simulink model "controladorNovo2015"  (R2015b)
settings: Solver=FixedStepDiscrete  SolverMode=SingleTasking  StartTime=0.0  StopTime=tmax  FixedStep=h  RelTol=1e-3
values from neighbouring files (symbols this model uses):
  G = [1; 1]    [init.m]    (also in initTemp.m = tf(N, D))
  h = 0.01    [init.m]    (also in initTemp.m)
  Qn = 0.01    [init.m]
  R = 0.01    [init.m]
  x0 = [1;1]    [init.m]
undefined symbols (not defined in the file or in its folder): C, Cd, gama, H, phi
libraries: simulink x1, dspsrcs4 x1
settings Model: Creator=Raposo  LastModifiedBy=lucasperovani
settings DataIOCC: LimitDataPoints=off
settings DebuggingCC: SFUnexpectedBacktrackingDiag=error  SFNoUnconditionalDefaultTransitionDiag=error
settings HardwareCC: ProdWordSize=32  ProdHWDeviceType=Specified
settings ModelReferenceCC: PropagateSignalLabelsOutOfModel=on
settings GRTTargetCC: TargetLangStandard=C99 (ISO)
settings ConfigComp: CovMetricSettings=dwe  CovHtmlReporting=off  CovSaveCumulativeToWorkspaceVar=off  CovSaveSingleToWorkspaceVar=off  CovModelRefEnable=Off  CovExternalEMLEnable=on

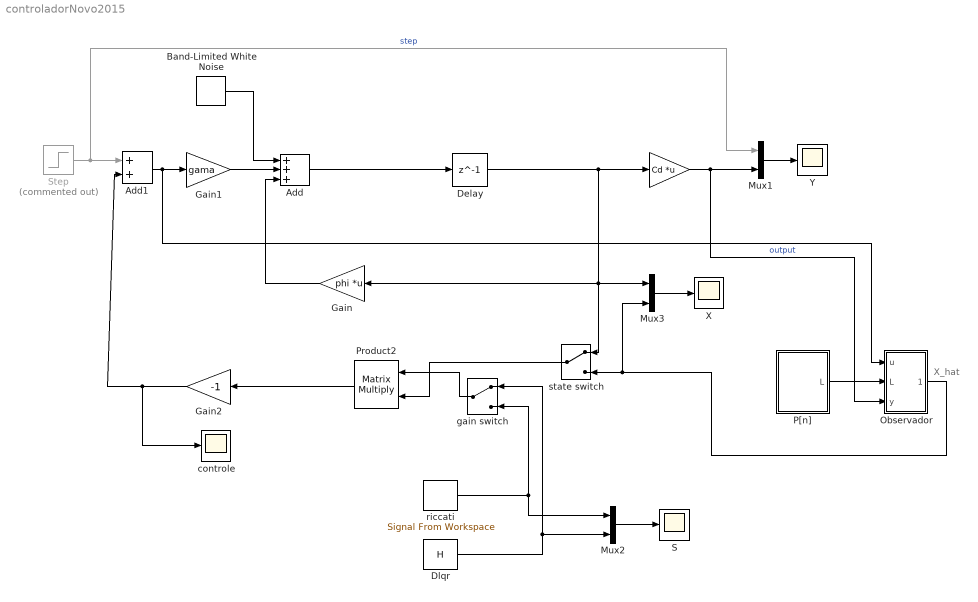
== system controladorNovo2015 ==
  note: X_hat
  " " : Gain  Gain=Cd  Multiplication=Matrix(K*u)
  Add : Sum  Inputs=+++
  Add1 : Sum
  Band-Limited White Noise : simulink/Sources/Band-Limited White Noise  Cov=[0.00000001]*0  Ts=h  seed=[23341]
  Delay : Delay  DelayLength=1  InitialCondition=x0  SampleTime=h
  Dlqr : Constant  Value=H  VectorParams1D=off
  Gain : Gain  Gain=phi  Multiplication=Matrix(K*u)
  Gain1 : Gain  Gain=gama
  Gain2 : Gain  Gain=-1
  Mux1 : Mux  Inputs=2
  Mux2 : Mux  Inputs=2
  Mux3 : Mux  Inputs=2
  "Observador " : Subsystem
  P[n] : Subsystem
  Product2 : Product  Multiplication=Matrix(*)
  S : Scope
  Step : Step  Commented=on  After=0  SampleTime=h
  X : Scope
  Y : Scope
  controle : Scope
  gain switch : ManualSwitch
  riccati : dspsrcs4/Signal From Workspace  X=lx'  Ts=1  nsamps=1  OutputAfterFinalValue=Setting to zero  ignoreOrWarnInputAndFrameLengths=off  OutputFrames=on
  state switch : ManualSwitch
  wires:
  Band-Limited White Noise/1 -> Add/1
  Gain/1 -> Add/3
  Delay/1 -> Mux3/1, state switch/1, Gain/1, " "/1
  riccati/1 -> Mux2/1, gain switch/2
  Step/1 -> Mux1/1, Add1/1  "step"
  Mux1/1 -> Y/1
  " "/1 -> "Observador "/3("y "), Mux1/2  "output"
  Mux2/1 -> S/1
  Add1/1 -> "Observador "/1(u), Gain1/1
  Gain1/1 -> Add/2
  Add/1 -> Delay/1
  Product2/1 -> Gain2/1
  Gain2/1 -> controle/1, Add1/2
  Dlqr/1 -> Mux2/2, gain switch/1
  gain switch/1 -> Product2/1
  P[n]/1(L) -> "Observador "/2(L)
  state switch/1 -> Product2/2
  "Observador "/1(Out1) -> Mux3/2, state switch/2
  Mux3/1 -> X/1

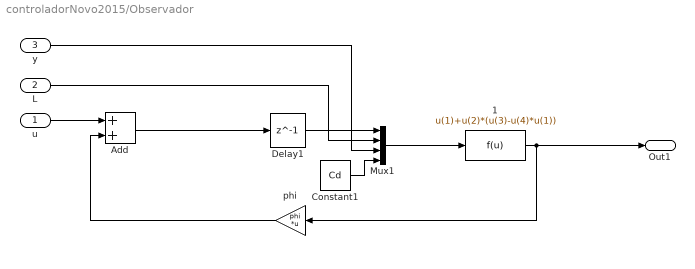
== system controladorNovo2015/Observador  ==
  u : Inport
  L : Inport  Port=2
  "y " : Inport  Port=3
  1 : Fcn  Expr=u(1)+u(2)*(u(3)-u(4)*u(1))
  Add : Sum
  Constant1 : Constant  Value=Cd  VectorParams1D=off
  Delay1 : Delay  DelayLength=1  InitialCondition=x0  SampleTime=h
  Mux1 : Mux
  phi : Gain  Gain=phi  Multiplication=Matrix(K*u)
  Out1 : Outport
  wires:
  phi/1 -> Add/2
  u/1 -> Add/1
  Add/1 -> Delay1/1
  Mux1/1 -> 1/1
  1/1 -> Out1/1, phi/1
  "y "/1 -> Mux1/3
  Delay1/1 -> Mux1/1
  L/1 -> Mux1/2
  Constant1/1 -> Mux1/4

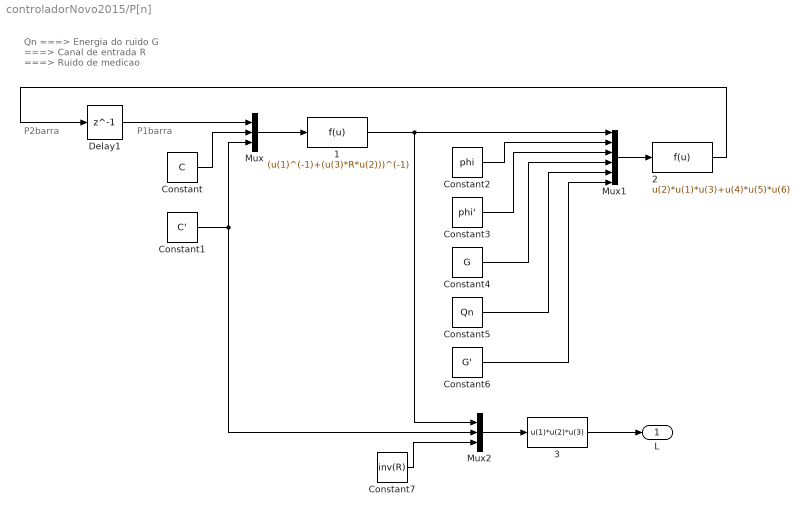
== system controladorNovo2015/P[n] ==
  note: Qn ===> Energia do ruido
      | G   ===> Canal de entrada
      | R   ===> Ruido de medicao
  note: P2barra
  note: P1barra
  1 : Fcn  Expr=(u(1)^(-1)+(u(3)*R*u(2)))^(-1)
  2 : Fcn  Expr=u(2)*u(1)*u(3)+u(4)*u(5)*u(6)
  3 : Fcn  Expr=u(1)*u(2)*u(3)
  Constant : Constant  Value=C  VectorParams1D=off
  Constant1 : Constant  Value=C'  VectorParams1D=off
  Constant2 : Constant  Value=phi  VectorParams1D=off
  Constant3 : Constant  Value=phi'  VectorParams1D=off
  Constant4 : Constant  Value=G  VectorParams1D=off
  Constant5 : Constant  Value=Qn  VectorParams1D=off
  Constant6 : Constant  Value=G'  VectorParams1D=off
  Constant7 : Constant  Value=inv(R)  VectorParams1D=off
  Delay1 : Delay  DelayLength=1  InitialCondition=0
  Mux : Mux  Inputs=3
  Mux1 : Mux  Inputs=6
  Mux2 : Mux  Inputs=3
  L : Outport
  wires:
  1/1 -> Mux2/1, Mux1/1
  2/1 -> Delay1/1
  3/1 -> L/1
  Delay1/1 -> Mux/1
  Mux/1 -> 1/1
  Constant/1 -> Mux/2
  Constant1/1 -> Mux2/2, Mux/3
  Mux1/1 -> 2/1
  Constant2/1 -> Mux1/2
  Constant3/1 -> Mux1/3
  Constant4/1 -> Mux1/4
  Constant5/1 -> Mux1/5
  Constant6/1 -> Mux1/6
  Mux2/1 -> 3/1
  Constant7/1 -> Mux2/3
